simulink model "bluetooth_voice"  (Simulink 6.0)
settings: Solver=ode3  SolverMode=SingleTasking  StartTime=0.0  StopTime=2.7  RelTol=1e-3
PreLoadFcn:
  | bluetooth_init;
PostLoadFcn:
  | bluetooth_cb
values from neighbouring files (symbols this model uses):
  Access_Code = zeros(72,1); Access_Code(1:2:72)=1    [bluetooth_init.m]
  ARQ = [1]    [bluetooth_init.m]
  awgn_802_seed = randseed(3)    [bluetooth_init.m]
  awgn_channel_seed = randseed(2)    [bluetooth_init.m]
  data_seed = randseed(5)    [bluetooth_init.m]
  Flow_Control = [1]    [bluetooth_init.m]
  HV_Type = 3    [bluetooth_cb.m]
  Input_Fs = 8000    [bluetooth_init.m]
  One_Zero_Payload = zeros(240,1)    [bluetooth_init.m]
  Packet_Type = [1 0 1 0]'    [bluetooth_init.m]
  rate_802_seed = randseed(4)    [bluetooth_init.m]
  Sequence = [1]    [bluetooth_init.m]
  Slave_Address = [1 0 1]'    [bluetooth_init.m]
  Slot_Ts = (1/1600)    (= 0.000625)    [bluetooth_cb.m]
undefined symbols (not defined in the file or in its folder): figposition, Fs, jet, Num_Slots_Rate, slcm, Slot_Enable_Phase, Tx_Ts
libraries: commblkcod2 x48, dspsrcs4 x22, dspsigops x19, simulink x15, dspbuff3 x8, dspindex x7, dspsigattribs x6, dspmtrx3 x5, dsparch4 x4, commdigbbndfm2 x4, bluetooth_lib x4, dspsnks4 x4
(part 1 of 2)
CloseFcn:
  | % Clear model variables
  | clear ARQ   Access_Code   BER_Results   Flow_Control   HV_Type   Input_Fs
  | clear Num_802_packets   Num_Payload_Bits   Num_Slots_Rate   One_Zero_Payload
  | clear Packet_Type   Sequence   Slave_Address   Slot_Enable_Phase   Slot_Pair
  | clear Slot_Ts   Tx_Ts   awgn_802_seed   awgn_channel_seed   data_seed
  | clear fixed_hop_freq   hop_seed   interp_coeffs   rate_802_seed   sigin
  | clear sigout   bluetoothSigsOut   y
settings Model: Creator=Stuart McGarrity  LastModifiedBy=mmclerno  ExtModeAutoUpdateStatusClock=off  BufferReuse=off  ProdHWDeviceType=Specified
settings Model: ModifiedComment=|
  | stuartm -- Fri Jul 20 12:58:27 2001 -- Version 1.201
  | Fix for R12.1. Changed CPM modulator. Replaced enable subsystems in channel with "switch case".
settings DataIOCC: SaveOutput=off  SaveTime=off  SignalLoggingName=bluetoothSigsOut
settings OptimizationCC: BlockReduction=off  BooleanDataType=off  InlineInvariantSignals=off  OptimizeBlockIOStorage=off  BufferReuse=off  EnforceIntegerDowncast=off  ExpressionFolding=off  FoldNonRolledExpr=off  LocalBlockOutputs=off
settings DebuggingCC: SolverPrmCheckMsg=none  InheritedTsInSrcMsg=none
settings HardwareCC: ProdHWDeviceType=Specified
settings ModelReferenceCC: UpdateModelReferenceTargets=IfOutOfDate
settings CodeAppCC: MangleLength=5

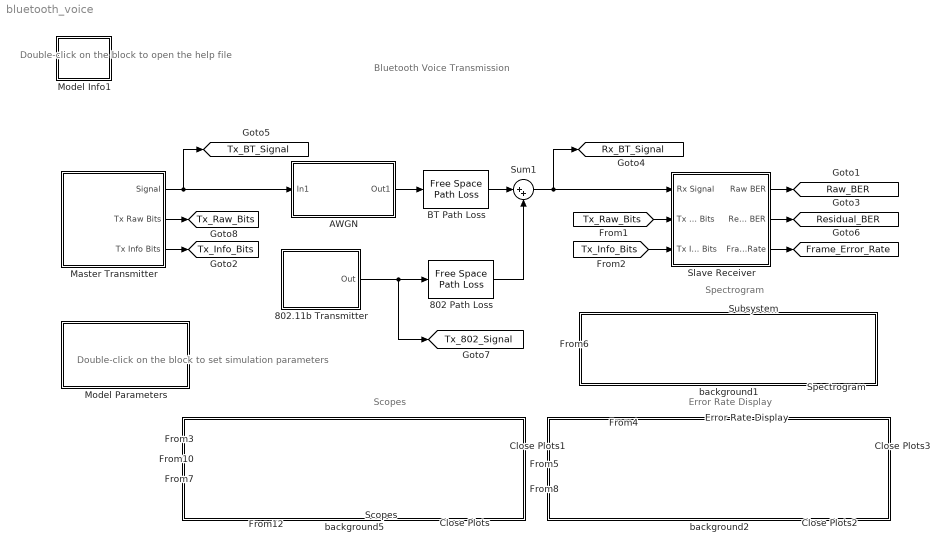
== system bluetooth_voice ==
  note: Bluetooth Voice Transmission
  note: Spectrogram
  note: Error Rate Display
  note: Scopes
  note: Double-click on the block
      | to open the help file
  note: Double-click on the block
      | to set simulation parameters
  802 Path Loss : commrflib2/Free Space Path Loss  mode=Decibels  dB=40  d=0.100  fc=1920
  802.11b Transmitter : Subsystem  AncestorBlock=bluetooth_lib/802.11b Transmitter  PropExecContextAcrossSSBoundary=on  mask{On=on, rate=200, m=1e-3, power=0.1, Freq_Number=39, rate_seed=rate_802_seed, awgn_seed=awgn_802_seed}
      mask prompts: On "Turn On 802.11"; rate "Average Rate (1/sec) (999 for constant)"; m "Length (secs)"; Freq_Number "Frequency Number (0-78)"; rate_seed "Rate Seed"; awgn_seed "Noise seed"
      mask init:
      | if On==1
      |    str='On';
      | else
      |   str='Off';
      | end;
      | 
      | adjusted_rate=rate/(1-rate*m); % account for finite packet length reducing rate
      mask Display: disp(['802.11b\nInterferer\n' str])
  AWGN : Subsystem  TreatAsAtomicUnit=on  PropExecContextAcrossSSBoundary=on  mask(Optional channel){AWGN_On=off, EsNo=15, Power=.001, Symbol_Period=1e-6, seed=awgn_channel_seed}
      mask prompts: AWGN_On "Turn on AWGN"; EsNo "Es/No"; Power "Input Power"; Symbol_Period "Symbol Period"
      mask init:
      | if AWGN_On==1
      |    Name='On';
      | else
      |   Name='Off';
      | end;
      mask Display: disp(['AWGN is ' Name])
  BT Path Loss : commrflib2/Free Space Path Loss  mode=Decibels  dB=40  d=0.100  fc=1920
  Close Plots : Subsystem  PropExecContextAcrossSSBoundary=on
      settings: OpenFcn=|
      | set_param([gcs,'/Scopes/State'],'Value','0');
      |   sdspfscope2([],[],[],'ScopeUpdate',[gcs '/Scopes/Subsystem/Timing Diagram'],'CloseFig');
      |   sdspfscope2([],[],[],'ScopeUpdate',[gcs '/Scopes/Subsystem/Spectrum Plot'],'CloseFig');
      | 
      | set_param([gcs '/Scopes/Subsystem/Timing Diagram'],'OpenScopeAtSimStart','off');
      | 
      | set_param([gcs '/Scopes/Subsystem/Spectrum Plot'],'OpenScopeAtSimStart','off');
      mask Display: disp('Close Scopes');
  Close Plots1 : Subsystem  PropExecContextAcrossSSBoundary=on
      settings: OpenFcn=|
      | set_param([gcs,'/Scopes/State'],'Value','1');
      |   sdspfscope2([],[],[],'ScopeUpdate',[gcs '/Scopes/Subsystem/Timing Diagram'],'OpenFig');
      |   sdspfscope2([],[],[],'ScopeUpdate',[gcs '/Scopes/Subsystem/Spectrum Plot'],'OpenFig');
      | 
      | set_param([gcs '/Scopes/Subsystem/Timing Diagram'],'OpenScopeAtSimStart','on');
      | 
      | set_param([gcs '/Scopes/Subsystem/Spectrum Plot'],'OpenScopeAtSimStart','on');
      mask Display: disp('Open Scopes');
  Close Plots2 : Subsystem  PropExecContextAcrossSSBoundary=on
      settings: OpenFcn=set_param([gcs '/Error Rate Display'],'Open','off');
      mask Display: disp('Close Scopes');
  Close Plots3 : Subsystem  PropExecContextAcrossSSBoundary=on
      settings: OpenFcn=set_param([gcs '/Error Rate Display'],'Open','on');
      mask Display: disp('Open Scopes');
  Error Rate Display : Subsystem  TreatAsAtomicUnit=on  PropExecContextAcrossSSBoundary=on
      mask Display: disp('Error\nRate\nDisplay')
  Master Transmitter : Subsystem  PropExecContextAcrossSSBoundary=on
      mask Type: Master Transmitter
      mask Display: plot(0,0,100,100,[30,60,60,55,55,30,30],[10,10,90,90,70,70,10],[35,35,55,55,35],[64,45,45,64,64])
  Model Info1 : Subsystem  LoadFcn=slcm LoadBlock;  InitFcn=slcm('UpdateAllCMBlocksInThisModelInit')  PropExecContextAcrossSSBoundary=on  mask(CMBlock){InitialSaveTempField=, InitialBlockCM=none, BlockCM=none, Frame=on, SaveTempField=, DisplayStringWithTags=Info, MaskDisplayString=Info, HorizontalTextAlignment=Center, LeftAlignmentValue=0.5, SourceBlockDiagram=bluetooth_voice, TagMaxNumber=20, CMTag1=, CMTag2=, CMTag3=, CMTag4=, CMTag5=, CMTag6=, CMTag7=, CMTag8=, CMTag9=, CMTag10=, CMTag11=, CMTag12=, CMTag13=, CMTag14=, CMTag15=, CMTag16=, CMTag17=, CMTag18=, CMTag19=, CMTag20=}
      mask help: This block allows revision control information to be displayed within the model.
      settings: CopyFcn=slcm CopyBlock;  DeleteFcn=slcm Cancel;  PostSaveFcn=slcm('UpdateAllCMBlocksInThisModel')  NameChangeFcn=slcm Rename;  OpenFcn=commdemohelp;
      mask Display: text(str2num(LeftAlignmentValue), 0.5, MaskDisplayString, 'HorizontalAlignment', HorizontalTextAlignment)
  Model Parameters : Subsystem  TreatAsAtomicUnit=on  PropExecContextAcrossSSBoundary=on  mask(Bluetooth Initial Settings ){HV_Type=HV3, Slot_Pair1=1&2, Slot_Pair2=5&6}
      mask prompts: HV_Type "HV Packet Type"; Slot_Pair1 "Initial Slot Pair for HV2"; Slot_Pair2 "Initial Slot Pair for HV3"
      mask help: Use the following mask to select different parameters for simulation.
      mask StyleString: popup(HV1|HV2|HV3),popup(1&2|3&4),popup(1&2|3&4|5&6)
      mask CallbackString: bluetooth_cb;||
      mask Display: disp('Double-click\n to select\n Model Parameters')
  Scopes : Subsystem  TreatAsAtomicUnit=on  PropExecContextAcrossSSBoundary=on
      mask Display: disp('Scopes')
  Slave Receiver : Subsystem  PropExecContextAcrossSSBoundary=on
      mask Type: Slave Receiver
      mask Display: plot(15,5,95,80,[26, 28,35,44,58,85,87,92,86,59,46,46,38, 31, 27,26],[55,49,45,45,34,15,10,16,17,37,50,58,66,67,62,55],[32,34,37,42,46,46],[67,69,71,70,66,58],[27,25,24,21,23,26],[52,49,45,47,52,58],[35,38,40,42,44],[66,67,66,64,61],[34,32,38,40,34],[60,56,51,55,60])
  Spectrogram : dspsnks4/Matrix Viewer  ImageParams=on  CMapStr=jet(256)  AxisColorbar=off  AxisParams=on  AxisOrigin=Lower left corner  XLabel=Time Index  YLabel=Frequency Index  ZLabel=dB Magnitude  FigPos=figposition([2.5 8.5 70 25]);  AxisZoom=on
      settings: YMin=-60  YMax=-30
  Subsystem : Subsystem  PropExecContextAcrossSSBoundary=on
      mask Display: disp('Rx_BT_Signal\nProcessing')
  Sum1 : Sum  Inputs=|++  SaturateOnIntegerOverflow=on  InputSameDT=on
  background1 : Subsystem  PropExecContextAcrossSSBoundary=on
      mask Display: disp('')
  background2 : Subsystem  PropExecContextAcrossSSBoundary=on
      mask Display: disp('')
  background5 : Subsystem  PropExecContextAcrossSSBoundary=on
      mask Display: disp('')
  tag scope: Frame_Error_Rate=global, Raw_BER=global, Residual_BER=global, Rx_BT_Signal=global, Tx_802_Signal=global, Tx_BT_Signal=global, Tx_Info_Bits=global, Tx_Raw_Bits=global
  wires:
  Sum1/1 -> [Rx_BT_Signal], Slave Receiver/1(Rx Signal)
  Master Transmitter/2(Tx Raw Bits) -> [Tx_Raw_Bits]
  [Tx_Raw_Bits] -> Slave Receiver/2(Tx Raw Bits)
  Master Transmitter/3(Tx Info Bits) -> [Tx_Info_Bits]
  [Tx_Info_Bits] -> Slave Receiver/3(Tx Info Bits)
  802.11b Transmitter/1(Out) -> [Tx_802_Signal], 802 Path Loss/1
  802 Path Loss/1 -> Sum1/2
  AWGN/1(Out1) -> BT Path Loss/1
  BT Path Loss/1 -> Sum1/1
  [Tx_BT_Signal] -> Scopes/1(Tx)
  [Rx_BT_Signal] -> Scopes/3(Rx)
  [Tx_802_Signal] -> Scopes/2(Tx_802)
  [Packet_Envelope_802] -> Scopes/4(Tx_802 Envelope)
  Master Transmitter/1(Signal) -> AWGN/1(In1), [Tx_BT_Signal]
  Slave Receiver/1(Raw BER) -> [Raw_BER]
  Slave Receiver/2(Residual BER) -> [Residual_BER]
  Slave Receiver/3(Frame Error Rate) -> [Frame_Error_Rate]
  [Raw_BER] -> Error Rate Display/1(Tx)
  [Residual_BER] -> Error Rate Display/2(Tx_802)
  [Frame_Error_Rate] -> Error Rate Display/3(Rx)
  Subsystem/1(Out1) -> Spectrogram/1
  [Rx_BT_Signal] -> Subsystem/1(In1)

== system bluetooth_voice/802.11b Transmitter ==
  1/100packet resolution : ZeroOrderHold  SampleTime=(1/1600)/100
  22MHz noise in 100MHz signal : Subsystem  TreatAsAtomicUnit=on  PropExecContextAcrossSSBoundary=on
  Buffer to same frame-size as channel : dspbuff3/Buffer  N=62500  V=0  ic=0
  Enable control : Subsystem  PropExecContextAcrossSSBoundary=on
      mask Display:
      | disp('Enable\n
      | Logic')
  Square pulse with Poisson process : Subsystem  PropExecContextAcrossSSBoundary=on  mask(Poisson process){rate=adjusted_rate, m=m, seed=rate_seed}
      mask prompts: rate "Average Rate (1/sec)"; m "Mean Length"
      mask Display: plot(exp(-(0:.4:3)))
  Out : Outport
  tag scope: Packet_Envelope_802=global
  wires:
  22MHz noise in 100MHz signal/1(Out) -> Buffer to same frame-size as channel/1
  Buffer to same frame-size as channel/1 -> Out/1
  1/100packet resolution/1 -> Enable control/1(In)
  Square pulse with Poisson process/1(hit) -> 1/100packet resolution/1, [Packet_Envelope_802]
  Enable control/1(Out) -> 22MHz noise in 100MHz signal/Enable

== system bluetooth_voice/AWGN ==
  In1 : Inport  LatchInput=off
  Generate noise only for slot 1 : simulink/Signal Routing/Manual Switch  sw=0  action=0
  Mode : Constant  Value=AWGN_On  SampleTime=Inf
  Slot 1 enable2 : dspsrcs4/Signal From Workspace  X=[1 0 0 0 0 0]  Ts=625e-6  nsamps=1  OutputAfterFinalValue=Cyclic repetition
  Slot 1 enable3 : dspsrcs4/Signal From Workspace  X=[1 1 1 1 1 1 ]  Ts=625e-6  nsamps=1  OutputAfterFinalValue=Cyclic repetition
  Subsystem : Subsystem  TreatAsAtomicUnit=on  PropExecContextAcrossSSBoundary=on
  Out1 : Outport  InitialOutput=0
  wires:
  Mode/1 -> Subsystem/1(In1)
  Subsystem/1(Out1) -> Out1/1
  Slot 1 enable3/1 -> Generate noise only for slot 1/2
  Generate noise only for slot 1/1 -> Subsystem/Enable
  Slot 1 enable2/1 -> Generate noise only for slot 1/1
  In1/1 -> Subsystem/2(In2)

== system bluetooth_voice/Close Plots ==

== system bluetooth_voice/Close Plots1 ==

== system bluetooth_voice/Close Plots2 ==

== system bluetooth_voice/Close Plots3 ==

== system bluetooth_voice/Error Rate Display ==
  note: Total number of bits
  note: Raw Bit Errors
  note: Raw BER
  note: Residual BER
  note: Residual Bit Error
  note: Total number of bits
  note: FER
  note: Frame Errors
  note: Total number of Frames
  Tx : Inport  LatchInput=off
  Tx_802 : Inport  Port=2  LatchInput=off
  Rx : Inport  Port=3  LatchInput=off
  FER Display : Display
  Raw BER Display : Display
  Residual BER Display : Display
  wires:
  Rx/1 -> FER Display/1
  Tx/1 -> Raw BER Display/1
  Tx_802/1 -> Residual BER Display/1

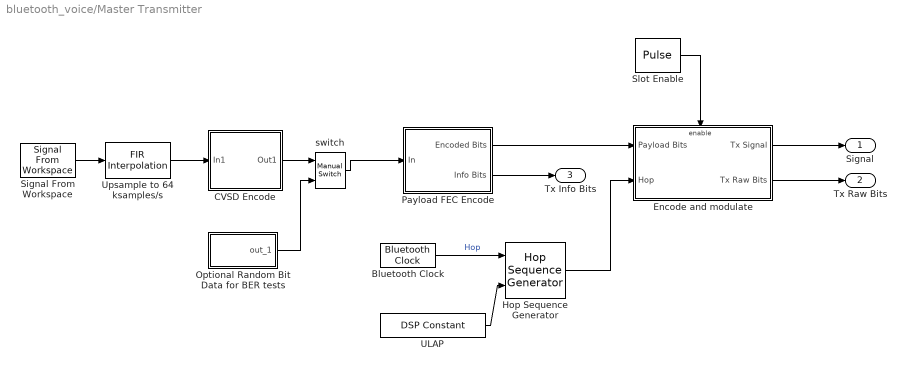
== system bluetooth_voice/Master Transmitter ==
  Bluetooth Clock : bluetooth_lib/Bluetooth Clock  Ts=(1/1600)/2
  CVSD Encode : Subsystem  PropExecContextAcrossSSBoundary=on  mask(CVSD Encoder){min_step=10, max_step=1280, accum_decay=1-1/32, step_decay=1-1/1024}
      mask prompts: min_step "Minimum Step Size"; max_step "Maximum Step Size"; accum_decay "Accumulator Decay"; step_decay "Step Decay"
      mask help: Encode a 64 K samples per sec speech signal into a 64Kbps bit stream.
      mask init:
      | pos_accum_max = 2^15 - 1;
      | neg_accum_max = -2^15 + 1;
      mask Display: disp('CVSD\nEncode')
  Encode and modulate : Subsystem  TreatAsAtomicUnit=on  PropExecContextAcrossSSBoundary=on
  Hop Sequence Generator : bluetooth_lib/Hop Sequence Generator  Hop_Mode=Connection State Hop Sequence  hop_seed=hop_seed  fixed_hop_freq=fixed_hop_freq
  Optional Random Bit Data for BER tests : Subsystem  PropExecContextAcrossSSBoundary=on  mask(Random-Integer Generator){mul=2, seed=data_seed, Ts=1/64000, frameBased=off, sampPerFrame=1, orient=off}
      mask prompts: mul "M-ary number:"; seed "Initial seed:"; Ts "Sample time:"; frameBased "Frame-based outputs"; sampPerFrame "Samples per frame:"; orient "Interpret vector parameters as 1-D"
      mask help: Generate integers randomly distributed in range [0, M-1], where M is the M-ary number.
      mask init:
      | if (frameBased & sampPerFrame > 1), dsp_sampFrame = sampPerFrame;
      | else dsp_sampFrame = 1; end
      | eStr=commblkrandintsrc2(gcb,'init');
      | if(eStr.ecode==1)
      |     error(eStr.emsg);
      | end
      mask Help: helpview(commbhelp)
      mask CallbackString: |||commblkrandintsrc2(gcb,'cbFrameBased');||commblkrandintsrc2(gcb,'cbOrient');
      mask Display: disp('Random bits')
  Payload FEC Encode : Subsystem  PropExecContextAcrossSSBoundary=on
  Signal From Workspace : dspsrcs4/Signal From Workspace  X=sigin  Ts=1/8000  nsamps=1  OutputAfterFinalValue=Setting to zero
  Slot Enable : DiscretePulseGenerator  Period=Num_Slots_Rate  PhaseDelay=Slot_Enable_Phase  SampleTime=Slot_Ts
  ULAP : dspsrcs4/DSP Constant  Value=hex2dec('2a96ef25')  SampleMode=Discrete  discreteOutput=Sample-based  continuousOutput=Sample-based  sampTime=(1/1600)/2  framePeriod=(1/1600)/2  dataType=Inherit from 'Constant value'  isSigned=on  wordLen=16  udDataType=sfix(16)  fracBitsMode=Best precision  numFracBits=15  InterpretAs1D=off  Ts=(1/1600)/2  FramebasedOutput=off
  Upsample to 64 ksamples/s : dspmlti3/FIR Interpolation  DialogController=dspDDGCreate  DialogControllerArgs=DataTag4  h=interp_coeffs  L=8  framing=Maintain input frame size  outputBufInitCond=0  roundingMode=Floor  overflowMode=off
  switch : simulink/Signal Routing/Manual Switch  sw=1  action=0
  Signal : Outport
  Tx Raw Bits : Outport  Port=2
  Tx Info Bits : Outport  Port=3
  wires:
  Slot Enable/1 -> Encode and modulate/Enable
  Encode and modulate/1(Tx Signal) -> Signal/1
  Payload FEC Encode/1(Encoded Bits) -> Encode and modulate/1(Payload Bits)
  Signal From Workspace/1 -> Upsample to 64 ksamples/s/1
  Payload FEC Encode/2(Info Bits) -> Tx Info Bits/1
  Encode and modulate/2(Tx Raw Bits) -> Tx Raw Bits/1
  Hop Sequence Generator/1 -> Encode and modulate/2(Hop)
  ULAP/1 -> Hop Sequence Generator/2
  Bluetooth Clock/1 -> Hop Sequence Generator/1  "Hop"
  Optional Random Bit Data for BER tests/1(out_1) -> switch/2
  CVSD Encode/1(Out1) -> switch/1
  switch/1 -> Payload FEC Encode/1(In)
  Upsample to 64 ksamples/s/1 -> CVSD Encode/1(In1)

== system bluetooth_voice/Model Info1 ==
  EmptySubsystem : Subsystem  PropExecContextAcrossSSBoundary=on

== system bluetooth_voice/Model Parameters ==

== system bluetooth_voice/Scopes ==
  Tx : Inport  LatchInput=off
  Tx_802 : Inport  Port=2  LatchInput=off
  Rx : Inport  Port=3  LatchInput=off
  Tx_802 Envelope : Inport  Port=4  LatchInput=off
  802.11 Packets  Transmitted : Display
  Counter : dspswit3/Counter  Direction=Up  CountEvent=Rising edge  CounterSize=User defined  MaxCount=1000  InitialCount=0  Output=Count  HitValue=32  ResetInput=off  SamplesPerFrame=1  Ts=1  CntDtype=double  HitDtype=Logical
  State : Constant
  Subsystem : Subsystem  TreatAsAtomicUnit=on  PropExecContextAcrossSSBoundary=on
  To Workspace : ToWorkspace  VariableName=Num_802_packets  SampleTime=-1  SaveFormat=Array
      settings: MaxDataPoints=1
  wires:
  Counter/1 -> To Workspace/1, 802.11 Packets  Transmitted/1
  State/1 -> Subsystem/Enable
  Tx_802 Envelope/1 -> Counter/1
  Tx_802/1 -> Subsystem/2(In2)
  Tx/1 -> Subsystem/1(In1)
  Rx/1 -> Subsystem/3(In3)

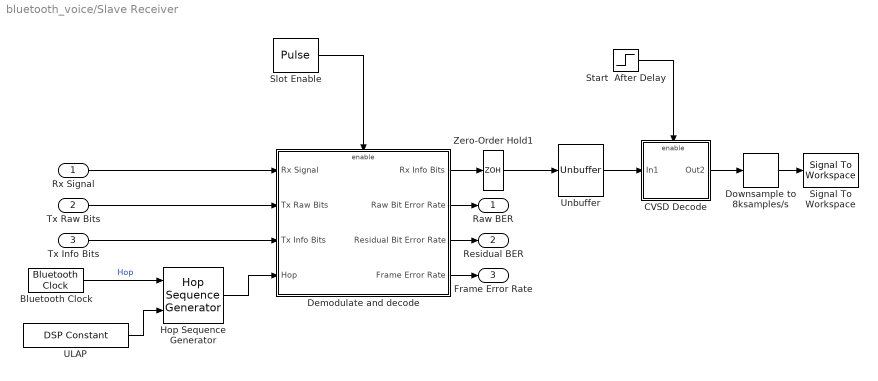
== system bluetooth_voice/Slave Receiver ==
  Rx Signal : Inport  LatchInput=off
  Tx Raw Bits : Inport  Port=2  LatchInput=off
  Tx Info Bits : Inport  Port=3  LatchInput=off
  Bluetooth Clock : bluetooth_lib/Bluetooth Clock  Ts=(1/1600)/2
  CVSD Decode : Subsystem  TreatAsAtomicUnit=on  PropExecContextAcrossSSBoundary=on  mask(CVSD Decoder){min_step=10, max_step=1280, accum_decay=1-1/32, step_decay=1-1/1024}
      mask prompts: min_step "Minimum Step Size"; max_step "Maximum Step Size"; accum_decay "Accumulator Decay"; step_decay "Step Decay"
      mask init:
      | pos_accum_max = 2^15 - 1;
      | neg_accum_max = -2^15 + 1;
      mask Display: disp('CVSD\nDecoder')
  Demodulate and decode : Subsystem  TreatAsAtomicUnit=on  PropExecContextAcrossSSBoundary=on
  Downsample to 8ksamples/s : dspsigops/Downsample  N=8  phase=0  ic=0  smode=Allow multirate  fmode=Maintain input frame size
  Hop Sequence Generator : bluetooth_lib/Hop Sequence Generator  Hop_Mode=Connection State Hop Sequence  hop_seed=hop_seed  fixed_hop_freq=fixed_hop_freq
  Signal To Workspace : dspsnks4/Signal To Workspace  VariableName=sigout  FrameMode=Concatenate frames (2-D array)
      settings: FixptAsFi=off
  Slot Enable : DiscretePulseGenerator  Period=Num_Slots_Rate  PhaseDelay=Slot_Enable_Phase  SampleTime=Slot_Ts
  Start  After Delay : Step  Time=0.01  SampleTime=1/64000
  ULAP : dspsrcs4/DSP Constant  Value=hex2dec('2a96ef25')  SampleMode=Discrete  discreteOutput=Sample-based  continuousOutput=Sample-based  sampTime=(1/1600)/2  framePeriod=(1/1600)/2  dataType=Inherit from 'Constant value'  isSigned=on  wordLen=16  udDataType=sfix(16)  fracBitsMode=Best precision  numFracBits=15  InterpretAs1D=off  Ts=(1/1600)/2  FramebasedOutput=off
  Unbuffer : dspbuff3/Unbuffer  ic=0
  Zero-Order Hold1 : ZeroOrderHold  SampleTime=Tx_Ts
  Raw BER : Outport  InitialOutput=0
  Residual BER : Outport  Port=2  InitialOutput=0
  Frame Error Rate : Outport  Port=3  InitialOutput=0
  wires:
  Slot Enable/1 -> Demodulate and decode/Enable
  Rx Signal/1 -> Demodulate and decode/1(Rx Signal)
  Tx Raw Bits/1 -> Demodulate and decode/2(Tx Raw Bits)
  CVSD Decode/1(Out2) -> Downsample to 8ksamples/s/1
  Demodulate and decode/1(Rx Info Bits) -> Zero-Order Hold1/1
  ULAP/1 -> Hop Sequence Generator/2
  Bluetooth Clock/1 -> Hop Sequence Generator/1  "Hop"
  Hop Sequence Generator/1 -> Demodulate and decode/4(Hop)
  Zero-Order Hold1/1 -> Unbuffer/1
  Start  After Delay/1 -> CVSD Decode/Enable
  Unbuffer/1 -> CVSD Decode/1(In1)
  Tx Info Bits/1 -> Demodulate and decode/3(Tx Info Bits)
  Demodulate and decode/3(Residual Bit Error Rate) -> Residual BER/1
  Demodulate and decode/2(Raw Bit Error Rate) -> Raw BER/1
  Demodulate and decode/4(Frame Error Rate) -> Frame Error Rate/1
  Downsample to 8ksamples/s/1 -> Signal To Workspace/1

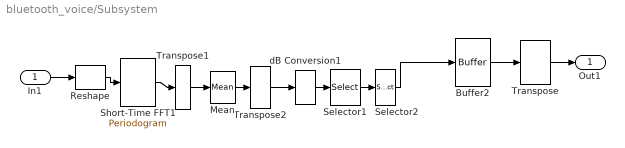
== system bluetooth_voice/Subsystem ==
  In1 : Inport  LatchInput=off
  Buffer2 : dspbuff3/Buffer  N=60  V=59  ic=-70
  Mean : dspstat3/Mean  DialogController=dspDDGCreate  DialogControllerArgs=DataTag8  run=off  reset_popup=None  roundingMode=Floor  overflowMode=off
  Reshape : simulink/Math Operations/Reshape  OutputDimensionality=Customize  OutputDimensions=[500,125]
  Selector1 : Selector  Elements=[257:512 1:256]  InputPortWidth=512
  Selector2 : Selector  Elements=7:506  InputPortWidth=512
  Short-Time FFT1 : dspspect3/Periodogram  wintype=Hanning  Rs=50  beta=5  winsamp=Periodic  inheritFFT=off  fftsize=512  navg=1
  Transpose : dspmtrx3/Transpose  Hermitian=off  overflowFlag=on
  Transpose1 : dspmtrx3/Transpose  Hermitian=off  overflowFlag=on
  Transpose2 : dspmtrx3/Transpose  Hermitian=off  overflowFlag=on
  dB Conversion1 : dspmathops/dB Conversion  dBtype=dB  intype=Power  R=1  fuzz=on
  Out1 : Outport
  wires:
  Selector2/1 -> Buffer2/1
  Selector1/1 -> Selector2/1
  Buffer2/1 -> Transpose/1
  Transpose2/1 -> dB Conversion1/1
  Transpose1/1 -> Mean/1
  Mean/1 -> Transpose2/1
  Reshape/1 -> Short-Time FFT1/1
  Short-Time FFT1/1 -> Transpose1/1
  dB Conversion1/1 -> Selector1/1
  Transpose/1 -> Out1/1
  In1/1 -> Reshape/1

== system bluetooth_voice/background1 ==

== system bluetooth_voice/background2 ==

== system bluetooth_voice/background5 ==

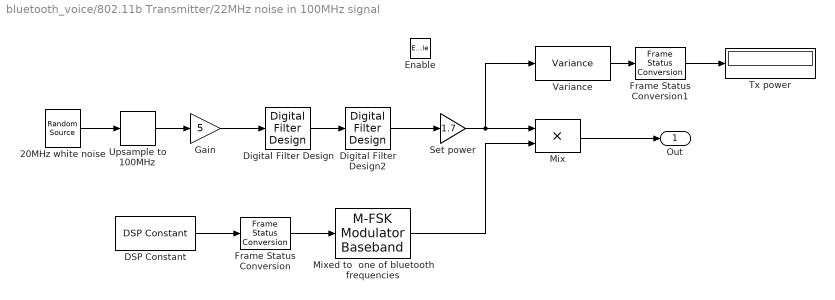
== system bluetooth_voice/802.11b Transmitter/22MHz noise in 100MHz signal ==
  Enable : EnablePort
  20MHz white noise : dspsrcs4/Random Source  SrcType=Gaussian  NormMethod=Ziggurat  CltLength=12  Min=0  Max=1  Mean=0  Var=power  RepMode=Specify seed  rawSeed=awgn_seed  Inherit=off  SampMode=Discrete  SampTime=1/20e6  SampFrame=62500/500  DataType=Double  OutComplex=Complex
  DSP Constant : dspsrcs4/DSP Constant  Value=Freq_Number  SampleMode=Discrete  discreteOutput=Sample-based  continuousOutput=Sample-based  sampTime=.01/1600  framePeriod=.01/1600  dataType=Inherit from 'Constant value'  isSigned=on  wordLen=16  udDataType=sfix(16)  fracBitsMode=Best precision  numFracBits=15  InterpretAs1D=off  Ts=.01/1600  FramebasedOutput=off
  Digital Filter Design : dsparch4/Digital Filter Design
  Digital Filter Design2 : dsparch4/Digital Filter Design
  Frame Status Conversion : dspsigattribs/Frame Status Conversion  growRefPort=off  outframe=Frame-based
  Frame Status Conversion1 : dspsigattribs/Frame Status Conversion  growRefPort=off  outframe=Sample-based
  Gain : Gain  Gain=5  SaturateOnIntegerOverflow=on
  Mix : Product  SaturateOnIntegerOverflow=on  InputSameDT=on
  "Mixed to  one of bluetooth frequencies " : commdigbbndfm2/M-FSK Modulator Baseband  M=79  InType=Integer  Enc=Binary  freqSep=1e6  phaseType=Continuous  numSamp=6.25e4/100
  Set power : Gain  Gain=1.7  SaturateOnIntegerOverflow=on
  Tx power : Display
  Upsample to 100MHz : dspsigops/Upsample  N=5  phase=0  ic=0  mode=Maintain input frame rate
  Variance : dspstat3/Variance  DialogController=dspDDGCreate  DialogControllerArgs=DataTag3  run=off  reset_popup=None  roundingMode=Floor  overflowMode=off
  Out : Outport  OutputWhenDisabled=reset  InitialOutput=0
  wires:
  Upsample to 100MHz/1 -> Gain/1
  Mix/1 -> Out/1
  20MHz white noise/1 -> Upsample to 100MHz/1
  Frame Status Conversion/1 -> "Mixed to  one of bluetooth frequencies "/1
  "Mixed to  one of bluetooth frequencies "/1 -> Mix/2
  DSP Constant/1 -> Frame Status Conversion/1
  Gain/1 -> Digital Filter Design/1
  Variance/1 -> Frame Status Conversion1/1
  Frame Status Conversion1/1 -> Tx power/1
  Set power/1 -> Mix/1, Variance/1
  Digital Filter Design2/1 -> Set power/1
  Digital Filter Design/1 -> Digital Filter Design2/1

== system bluetooth_voice/802.11b Transmitter/Enable control ==
  In : Inport  LatchInput=off
  If rate set to 999 turn-on always : RelationalOperator  Operator===  InputSameDT=on
  Logical Operator : Logic
  Logical Operator1 : Logic
  Logical Operator2 : Logic  Operator=OR
  Mode : Constant  Value=On
  Mode1 : Constant  Value=rate
  Mode2 : Constant  Value=999
  Out : Outport
  wires:
  Mode2/1 -> If rate set to 999 turn-on always/2
  Mode1/1 -> If rate set to 999 turn-on always/1
  If rate set to 999 turn-on always/1 -> Logical Operator1/2
  Logical Operator/1 -> Logical Operator2/1
  Mode/1 -> Logical Operator/2, Logical Operator1/1
  Logical Operator1/1 -> Logical Operator2/2
  In/1 -> Logical Operator/1
  Logical Operator2/1 -> Out/1

== system bluetooth_voice/802.11b Transmitter/Square pulse with Poisson process ==
  Abs : Abs  SaturateOnIntegerOverflow=on
  Derivative : Derivative
  Poisson Integer Generator : commrandsrc2/Poisson Integer Generator  lambda=adjusted_rate*m  seed=rate_seed  Ts=m  frameBased=off  sampPerFrame=1  orient=off
  Saturation : Saturate  UpperLimit=1  LowerLimit=0
  Zero-Order Hold : ZeroOrderHold  SampleTime=1e-3
  hit : Outport  InitialOutput=0
  wires:
  Poisson Integer Generator/1 -> Derivative/1
  Derivative/1 -> Saturation/1
  Abs/1 -> Zero-Order Hold/1
  Saturation/1 -> Abs/1
  Zero-Order Hold/1 -> hit/1

== system bluetooth_voice/AWGN/Subsystem ==
  In1 : Inport  LatchInput=off
  In2 : Inport  Port=2  LatchInput=off
  Enable : EnablePort
  Add noise : Subsystem  TreatAsAtomicUnit=on  PropExecContextAcrossSSBoundary=on
  If : If  IfExpression=u1 == 0
  Merge : Merge
  Pass Through : Subsystem  TreatAsAtomicUnit=on  PropExecContextAcrossSSBoundary=on
  Out1 : Outport
  wires:
  Add noise/1(Out1) -> Merge/2
  Pass Through/1(Out1) -> Merge/1
  If/1 -> Pass Through/Action
  In2/1 -> Pass Through/1(In1), Add noise/1(In1)
  If/2 -> Add noise/Action
  In1/1 -> If/1
  Merge/1 -> Out1/1

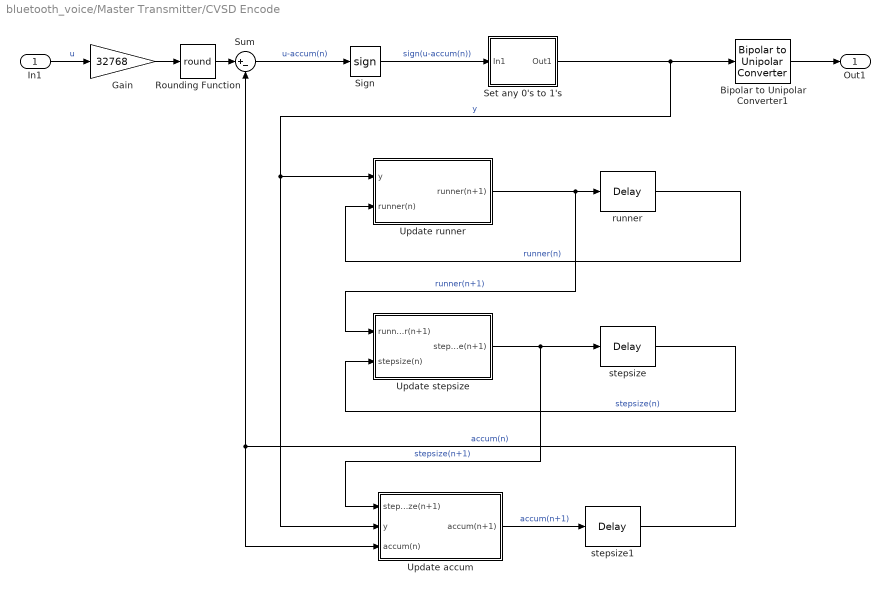
== system bluetooth_voice/Master Transmitter/CVSD Encode ==
  In1 : Inport  LatchInput=off
  Bipolar to Unipolar Converter1 : commutil2/Bipolar to Unipolar Converter  M=2  polarity=Negative
  Gain : Gain  Gain=32768  SaturateOnIntegerOverflow=on
  Rounding Function : Rounding  Operator=round
  Set any 0's to 1's : Subsystem  PropExecContextAcrossSSBoundary=on
  Sign : Signum
  Sum : Sum  Inputs=|+-  SaturateOnIntegerOverflow=on  InputSameDT=on
  Update accum : Subsystem  PropExecContextAcrossSSBoundary=on
  Update runner : Subsystem  PropExecContextAcrossSSBoundary=on
  Update stepsize : Subsystem  PropExecContextAcrossSSBoundary=on
  runner : dspsigops/Delay  dly_unit=Samples  delay=1  ic_detail=on  dif_ic_for_ch=off  dif_ic_for_dly=off  ic=10  reset_popup=None
  stepsize : dspsigops/Delay  dly_unit=Samples  delay=1  ic_detail=on  dif_ic_for_ch=off  dif_ic_for_dly=off  ic=min_step  reset_popup=None
  stepsize1 : dspsigops/Delay  dly_unit=Samples  delay=1  ic_detail=on  dif_ic_for_ch=off  dif_ic_for_dly=off  ic=min_step  reset_popup=None
  Out1 : Outport
  wires:
  Gain/1 -> Rounding Function/1
  Rounding Function/1 -> Sum/1
  Bipolar to Unipolar Converter1/1 -> Out1/1
  In1/1 -> Gain/1  "u"
  Sum/1 -> Sign/1  "u-accum(n)"
  stepsize1/1 -> Sum/2, Update accum/3(accum(n))  "accum(n)"
  Set any 0's to 1's/1(Out1) -> Bipolar to Unipolar Converter1/1, Update runner/1(y), Update accum/2(y)  "y"
  runner/1 -> Update runner/2(runner(n))  "runner(n)"
  Update runner/1(runner(n+1)) -> Update stepsize/1(runner(n+1)), runner/1  "runner(n+1)"
  Sign/1 -> Set any 0's to 1's/1(In1)  "sign(u-accum(n))"
  stepsize/1 -> Update stepsize/2(stepsize(n))  "stepsize(n)"
  Update stepsize/1(stepsize(n+1)) -> Update accum/1(stepsize(n+1)), stepsize/1  "stepsize(n+1)"
  Update accum/1(accum(n+1)) -> stepsize1/1  "accum(n+1)"

== system bluetooth_voice/Master Transmitter/Encode and modulate ==
  note: Framing: Bluetooth spec page 47
      | HEC: Bluetooth spec page 72
  Payload Bits : Inport  SampleTime=625e-6  LatchInput=off
  Hop : Inport  Port=2  SampleTime=625e-6  LatchInput=off
  Enable : EnablePort
  Access Code : dspsrcs4/DSP Constant  Value=Access_Code  SampleMode=Discrete  discreteOutput=Frame-based  continuousOutput=Sample-based  sampTime=Slot_Ts  framePeriod=Slot_Ts  dataType=Inherit from 'Constant value'  isSigned=on  wordLen=16  udDataType=sfix(16)  fracBitsMode=Best precision  numFracBits=15  InterpretAs1D=off  Ts=Slot_Ts  FramebasedOutput=on
  "Concatenate Access, Header and Payload" : simulink/Math Operations/Matrix Concatenation  numInports=3  catMethod=Vertical
  GFSK Modulate and frequency hop : Subsystem  PropExecContextAcrossSSBoundary=on
  General CRC Generator : commcrc2/General CRC Generator  genPoly=[1 1 0 1 0 0 1 1 1]  iniStates=[1 0 0 1 0 1 1 0]  numChecksums=1
  Header Info : Subsystem  PropExecContextAcrossSSBoundary=on
      mask Display: disp('Header Info')
  Header Info FEC Encode : dspsigops/Repeat  N=3  ic=0  mode=Maintain input frame rate
  Tx Signal : Outport  OutputWhenDisabled=reset  InitialOutput=0
  Tx Raw Bits : Outport  Port=2  OutputWhenDisabled=reset  InitialOutput=0
  wires:
  GFSK Modulate and frequency hop/1(Tx SIgnal) -> Tx Signal/1
  "Concatenate Access, Header and Payload"/1 -> GFSK Modulate and frequency hop/1(Tx Raw Bits), Tx Raw Bits/1
  General CRC Generator/1 -> Header Info FEC Encode/1  "HEC"
  Header Info/1(Out) -> General CRC Generator/1  "Header Info"
  Header Info FEC Encode/1 -> "Concatenate Access, Header and Payload"/2  "Header"
  Access Code/1 -> "Concatenate Access, Header and Payload"/1  "Access Code"
  Payload Bits/1 -> "Concatenate Access, Header and Payload"/3
  Hop/1 -> GFSK Modulate and frequency hop/2(Hop)

== system bluetooth_voice/Master Transmitter/Optional Random Bit Data for BER tests ==
  Frame Status Conversion : dspsigattribs/Frame Status Conversion  growRefPort=off  outframe=Sample-based
  Random Source : dspsrcs4/Random Source  SrcType=Uniform  NormMethod=Ziggurat  CltLength=12  Min=-1+eps  Max=mul-1  Mean=0  Var=1  RepMode=Specify seed  rawSeed=seed  Inherit=off  SampMode=Discrete  SampTime=Ts  SampFrame=dsp_sampFrame  DataType=Double  OutComplex=Real
  Reshape : simulink/Math Operations/Reshape  OutputDimensionality=1-D array  OutputDimensions=[sampPerFrame,max([length(mul), length(seed)])]
  Rounding Function : Rounding  Operator=ceil
  out_1 : Outport  InitialOutput=0
  wires:
  Frame Status Conversion/1 -> Reshape/1
  Random Source/1 -> Rounding Function/1
  Reshape/1 -> out_1/1
  Rounding Function/1 -> Frame Status Conversion/1

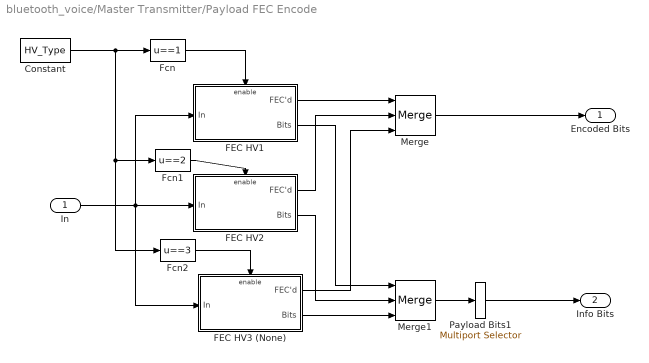
== system bluetooth_voice/Master Transmitter/Payload FEC Encode ==
  In : Inport  LatchInput=off
  Constant : Constant  Value=HV_Type
  FEC HV1 : Subsystem  TreatAsAtomicUnit=on  PropExecContextAcrossSSBoundary=on
  FEC HV2 : Subsystem  TreatAsAtomicUnit=on  PropExecContextAcrossSSBoundary=on
  FEC HV3 (None) : Subsystem  TreatAsAtomicUnit=on  PropExecContextAcrossSSBoundary=on
  Fcn : Fcn  Expr=u==1
  Fcn1 : Fcn  Expr=u==2
  Fcn2 : Fcn  Expr=u==3
  Merge : Merge  Inputs=3
  Merge1 : Merge  Inputs=3
  Payload Bits1 : dspindex/Multiport Selector  rowsOrCols=Rows  idxCellArray={1:Num_Payload_Bits}  idxErrMode=Clip Index
  Encoded Bits : Outport
  Info Bits : Outport  Port=2
  wires:
  In/1 -> FEC HV2/1(In), FEC HV1/1(In), FEC HV3 (None)/1(In)
  Constant/1 -> Fcn/1, Fcn1/1, Fcn2/1
  Fcn/1 -> FEC HV1/Enable
  Fcn1/1 -> FEC HV2/Enable
  Fcn2/1 -> FEC HV3 (None)/Enable
  FEC HV2/1(FEC'd) -> Merge/2
  FEC HV1/2(Bits) -> Merge1/1
  FEC HV2/2(Bits) -> Merge1/2
  FEC HV1/1(FEC'd) -> Merge/1
  Merge/1 -> Encoded Bits/1
  Merge1/1 -> Payload Bits1/1
  FEC HV3 (None)/1(FEC'd) -> Merge/3
  FEC HV3 (None)/2(Bits) -> Merge1/3
  Payload Bits1/1 -> Info Bits/1

== system bluetooth_voice/Model Info1/EmptySubsystem ==

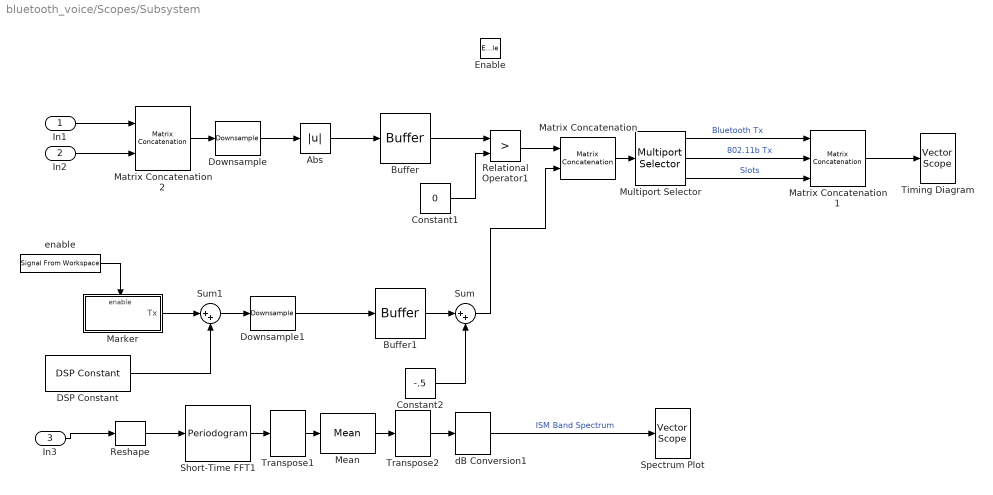
== system bluetooth_voice/Scopes/Subsystem ==
  In1 : Inport  LatchInput=off
  In2 : Inport  Port=2  LatchInput=off
  In3 : Inport  Port=3  LatchInput=off
  Enable : EnablePort
  Abs : Abs  SaturateOnIntegerOverflow=on
  Buffer : dspbuff3/Buffer  N=60*500  V=59*500  ic=0
  Buffer1 : dspbuff3/Buffer  N=60*500  V=59*500  ic=0
  Constant1 : Constant  Value=0
  Constant2 : Constant  Value=-.5
  DSP Constant : dspsrcs4/DSP Constant  Value=.2*[ones(1,36600) zeros(1,62500-36600)]'  SampleMode=Discrete  discreteOutput=Frame-based  continuousOutput=Sample-based  sampTime=625e-6  framePeriod=625e-6  dataType=Inherit from 'Constant value'  isSigned=on  wordLen=16  udDataType=sfix(16)  fracBitsMode=Best precision  numFracBits=15  InterpretAs1D=off  Ts=625e-6  FramebasedOutput=on
  Downsample : dspsigops/Downsample  N=125  phase=0  ic=0  smode=Allow multirate  fmode=Maintain input frame rate
  Downsample1 : dspsigops/Downsample  N=125  phase=0  ic=0  smode=Allow multirate  fmode=Maintain input frame rate
  Marker : Subsystem  TreatAsAtomicUnit=on  PropExecContextAcrossSSBoundary=on
  Matrix Concatenation : simulink/Math Operations/Matrix Concatenation  numInports=2  catMethod=Horizontal
  Matrix Concatenation1 : simulink/Math Operations/Matrix Concatenation  numInports=3  catMethod=Horizontal
  Matrix Concatenation2 : simulink/Math Operations/Matrix Concatenation  numInports=2  catMethod=Horizontal
  Mean : dspstat3/Mean  DialogController=dspDDGCreate  DialogControllerArgs=DataTag5  run=off  reset_popup=None  roundingMode=Floor  overflowMode=off
  Multiport Selector : dspindex/Multiport Selector  rowsOrCols=Columns  idxCellArray={ 1,2,3}  idxErrMode=Clip Index
  Relational Operator1 : RelationalOperator  Operator=>  InputSameDT=on
  Reshape : simulink/Math Operations/Reshape  OutputDimensionality=Customize  OutputDimensions=[500,125]
  Short-Time FFT1 : dspspect3/Periodogram  wintype=Hanning  Rs=50  beta=5  winsamp=Periodic  inheritFFT=off  fftsize=512  navg=1
  Spectrum Plot : dspsnks4/Vector Scope  ScopeProperties=off  Domain=Frequency  HorizSpan=1  DisplayProperties=off  AxisGrid=on  Memory=off  FrameNumber=on  AxisLegend=on  AxisZoom=off  OpenScopeAtSimStart=on  OpenScopeImmediately=off  FigPos=figposition([2.5 68.5 70 25]);  AxisProperties=off  XUnits=Hertz  XRange=[-Fs/2...Fs/2]  InheritXIncr=off  XIncr=1e-8  XLabel=Time  YUnits=Magnitude  YLabel=Magnitude, dB  LineProperties=off  LineStyles=--  LineColors=m
      settings: YMin=-80.906815143504  YMax=-25.7732682054945
  Sum : Sum  Inputs=|++  SaturateOnIntegerOverflow=on  InputSameDT=on
  Sum1 : Sum  Inputs=|++  SaturateOnIntegerOverflow=on  InputSameDT=on
  Timing Diagram : dspsnks4/Vector Scope  ScopeProperties=off  Domain=User-defined  HorizSpan=1  DisplayProperties=off  AxisGrid=on  Memory=off  FrameNumber=on  AxisLegend=on  AxisZoom=off  OpenScopeAtSimStart=on  OpenScopeImmediately=off  FigPos=figposition([2.5 37.5 70 25]);  AxisProperties=off  XUnits=Hertz  XRange=[0...Fs/2]  InheritXIncr=off  XIncr=125*1e-8  XLabel=Time (s)  YUnits=dB  YLabel=Amplitude  LineProperties=off  LineStyles=-|-  LineColors=[0 0 1]|[1 0 0]
      settings: YMin=-0.525  YMax=1.05
  Transpose1 : dspmtrx3/Transpose  Hermitian=off  overflowFlag=on
  Transpose2 : dspmtrx3/Transpose  Hermitian=off  overflowFlag=on
  dB Conversion1 : dspmathops/dB Conversion  dBtype=dB  intype=Power  R=1  fuzz=on
  enable : dspsrcs4/Signal From Workspace  X=[1 0 0 0 0 0]  Ts=625e-6  nsamps=1  OutputAfterFinalValue=Cyclic repetition
  wires:
  DSP Constant/1 -> Sum1/2
  Sum1/1 -> Downsample1/1
  Marker/1(Tx) -> Sum1/1
  Buffer1/1 -> Sum/1
  Constant2/1 -> Sum/2
  Matrix Concatenation/1 -> Multiport Selector/1
  Relational Operator1/1 -> Matrix Concatenation/1
  Sum/1 -> Matrix Concatenation/2
  Downsample1/1 -> Buffer1/1
  Multiport Selector/3 -> Matrix Concatenation1/3  "Slots"
  enable/1 -> Marker/Enable
  Multiport Selector/2 -> Matrix Concatenation1/2  "802.11b Tx"
  Multiport Selector/1 -> Matrix Concatenation1/1  "Bluetooth Tx"
  Matrix Concatenation2/1 -> Downsample/1
  In1/1 -> Matrix Concatenation2/1
  In2/1 -> Matrix Concatenation2/2
  Buffer/1 -> Relational Operator1/1
  Constant1/1 -> Relational Operator1/2
  Transpose2/1 -> dB Conversion1/1
  Transpose1/1 -> Mean/1
  Mean/1 -> Transpose2/1
  Reshape/1 -> Short-Time FFT1/1
  In3/1 -> Reshape/1
  Matrix Concatenation1/1 -> Timing Diagram/1
  Short-Time FFT1/1 -> Transpose1/1
  dB Conversion1/1 -> Spectrum Plot/1  "ISM Band Spectrum"
  Downsample/1 -> Abs/1
  Abs/1 -> Buffer/1

== system bluetooth_voice/Slave Receiver/CVSD Decode ==
  In1 : Inport  LatchInput=off
  Enable : EnablePort
  Delay : dspsigops/Delay  dly_unit=Samples  delay=1  ic_detail=on  dif_ic_for_ch=off  dif_ic_for_dly=off  ic=10  reset_popup=None
  Digital Filter Design : dsparch4/Digital Filter Design
  Gain1 : Gain  Gain=1/32768  SaturateOnIntegerOverflow=on
  Unipolar to Bipolar Converter : commutil2/Unipolar to Bipolar Converter  M=2  polarity=Negative
  Update accum : Subsystem  PropExecContextAcrossSSBoundary=on
  Update runner : Subsystem  PropExecContextAcrossSSBoundary=on
  Update stepsize : Subsystem  PropExecContextAcrossSSBoundary=on
  accum : dspsigops/Delay  dly_unit=Samples  delay=1  ic_detail=on  dif_ic_for_ch=off  dif_ic_for_dly=off  ic=0  reset_popup=None
  stepsize : dspsigops/Delay  dly_unit=Samples  delay=1  ic_detail=on  dif_ic_for_ch=off  dif_ic_for_dly=off  ic=min_step  reset_popup=None
  Out2 : Outport
  wires:
  In1/1 -> Unipolar to Bipolar Converter/1  "u"
  accum/1 -> Update accum/3(accum(n))  "accum(n)"
  Delay/1 -> Update runner/2(runner(n))  "runner(n)"
  Update runner/1(runner(n+1)) -> Update stepsize/1(runner(n+1)), Delay/1  "runner(n+1)"
  stepsize/1 -> Update stepsize/2(stepsize(n))  "stepsize(n)"
  Update stepsize/1(stepsize(n+1)) -> Update accum/1(stepsize(n+1)), stepsize/1  "stepsize(n+1)"
  Update accum/1(accum(n+1)) -> Gain1/1, accum/1  "accum(n+1)"
  Unipolar to Bipolar Converter/1 -> Update accum/2(u), Update runner/1(u)  "u"
  Digital Filter Design/1 -> Out2/1
  Gain1/1 -> Digital Filter Design/1

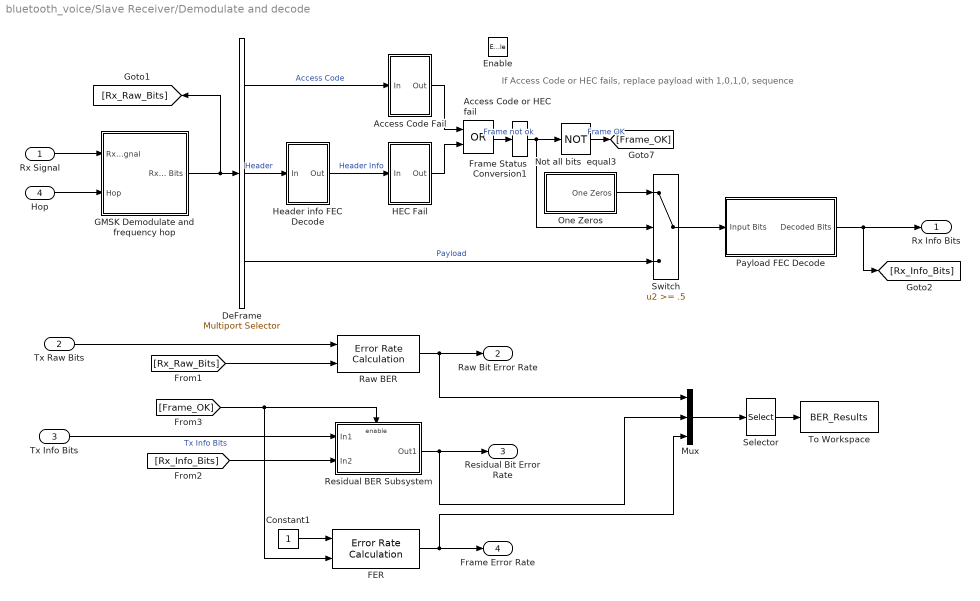
== system bluetooth_voice/Slave Receiver/Demodulate and decode ==
  note: If Access Code or HEC fails,
      | replace payload with 1,0,1,0, sequence
  Rx Signal : Inport  LatchInput=off
  Tx Raw Bits : Inport  Port=2  LatchInput=off
  Tx Info Bits : Inport  Port=3  LatchInput=off
  Hop : Inport  Port=4  SampleTime=Slot_Ts  LatchInput=off
  Enable : EnablePort
  Access Code Fail : Subsystem  PropExecContextAcrossSSBoundary=on
  Access Code or HEC fail : Logic  Operator=OR
  Constant1 : Constant
  DeFrame : dspindex/Multiport Selector  rowsOrCols=Rows  idxCellArray="{  1:72, 73:126,127:366}"  idxErrMode=Clip Index
  FER : commsink2/Error Rate Calculation  N=0  st_delay=0  cp_mode=Entire frame  subframe=[]  PMode=Port  WsName=ErrorVec  RsMode2=off  stop=on  numErr=100  maxBits=1e6
  Frame Status Conversion1 : dspsigattribs/Frame Status Conversion  growRefPort=off  outframe=Sample-based
  GMSK Demodulate and frequency hop : Subsystem  PropExecContextAcrossSSBoundary=on
  HEC Fail : Subsystem  PropExecContextAcrossSSBoundary=on
  Header info FEC Decode : Subsystem  PropExecContextAcrossSSBoundary=on
  Mux : Mux  Inputs=3
  Not all bits  equal3 : Logic  Operator=NOT  Inputs=1
  One Zeros : Subsystem  PropExecContextAcrossSSBoundary=on
  Payload FEC Decode : Subsystem  PropExecContextAcrossSSBoundary=on
  Raw BER : commsink2/Error Rate Calculation  N=0  st_delay=0  cp_mode=Entire frame  subframe=[]  PMode=Port  WsName=ErrorVec  RsMode2=off  stop=off  numErr=100  maxBits=1e6
  Residual BER Subsystem : Subsystem  TreatAsAtomicUnit=on  PropExecContextAcrossSSBoundary=on
  Selector : Selector  Elements=[1 4 7]  InputPortWidth=9
  Switch : Switch  Threshold=.5  InputSameDT=on
  To Workspace : ToWorkspace  VariableName=BER_Results  SampleTime=-1  SaveFormat=Array
      settings: MaxDataPoints=1
  Rx Info Bits : Outport  InitialOutput=0
  Raw Bit Error Rate : Outport  Port=2  InitialOutput=0
  Residual Bit Error Rate : Outport  Port=3  InitialOutput=0
  Frame Error Rate : Outport  Port=4  InitialOutput=0
  wires:
  Hop/1 -> GMSK Demodulate and frequency hop/2(Hop)
  Rx Signal/1 -> GMSK Demodulate and frequency hop/1(Rx Signal)
  Switch/1 -> Payload FEC Decode/1(Input Bits)
  Not all bits  equal3/1 -> [Frame_OK]  "Frame OK"
  Frame Status Conversion1/1 -> Not all bits  equal3/1, Switch/2
  HEC Fail/1(Out) -> Access Code or HEC fail/2
  Header info FEC Decode/1(Out) -> HEC Fail/1(In)  "Header Info"
  Access Code Fail/1(Out) -> Access Code or HEC fail/1
  Access Code or HEC fail/1 -> Frame Status Conversion1/1  "Frame not ok"
  DeFrame/2 -> Header info FEC Decode/1(In)  "Header"
  One Zeros/1(One Zeros) -> Switch/1
  DeFrame/1 -> Access Code Fail/1(In)  "Access Code"
  DeFrame/3 -> Switch/3  "Payload"
  Tx Info Bits/1 -> Residual BER Subsystem/1(In1)  "Tx Info Bits"
  [Rx_Info_Bits] -> Residual BER Subsystem/2(In2)
  Constant1/1 -> FER/1
  Selector/1 -> To Workspace/1
  Mux/1 -> Selector/1
  Raw BER/1 -> Mux/1, Raw Bit Error Rate/1
  Tx Raw Bits/1 -> Raw BER/1
  FER/1 -> Mux/3, Frame Error Rate/1
  [Frame_OK] -> FER/2, Residual BER Subsystem/Enable
  Residual BER Subsystem/1(Out1) -> Mux/2, Residual Bit Error Rate/1
  Payload FEC Decode/1(Decoded Bits) -> [Rx_Info_Bits], Rx Info Bits/1
  [Rx_Raw_Bits] -> Raw BER/2
  GMSK Demodulate and frequency hop/1(Rx Raw Bits) -> DeFrame/1, [Rx_Raw_Bits]

== system bluetooth_voice/AWGN/Subsystem/Add noise ==
  In1 : Inport  LatchInput=off
  Action Port : ActionPort  ActionType=else
  AWGN Channel1 : commchan2/AWGN Channel  seed=seed  noiseMode="Signal to noise ratio  (Es/No)"  EbNodB=10  EsNodB=EsNo  SNRdB=10  bitsPerSym=1  Ps=Power  Tsym=Symbol_Period  variance=1
  Out1 : Outport
  wires:
  In1/1 -> AWGN Channel1/1
  AWGN Channel1/1 -> Out1/1

== system bluetooth_voice/AWGN/Subsystem/Pass Through ==
  In1 : Inport  LatchInput=off
  Action Port : ActionPort  ActionType=then
  Out1 : Outport
  wires:
  In1/1 -> Out1/1

== system bluetooth_voice/Master Transmitter/CVSD Encode/Set any 0's to 1's ==
  In1 : Inport  LatchInput=off
  If : If  IfExpression=u1 ==0
  Merge : Merge
  Pass through : Subsystem  TreatAsAtomicUnit=on  PropExecContextAcrossSSBoundary=on
  Set to 1 : Subsystem  TreatAsAtomicUnit=on  PropExecContextAcrossSSBoundary=on
  Out1 : Outport
  wires:
  If/1 -> Set to 1/Action
  In1/1 -> Pass through/1(In1), If/1
  If/2 -> Pass through/Action
  Set to 1/1(1) -> Merge/1
  Pass through/1(Out1=In1) -> Merge/2
  Merge/1 -> Out1/1  "y"

== system bluetooth_voice/Master Transmitter/CVSD Encode/Update accum ==
  stepsize(n+1) : Inport  LatchInput=off
  y : Inport  Port=2  LatchInput=off
  accum(n) : Inport  Port=3  LatchInput=off
  Gain : Gain  Gain=accum_decay  SaturateOnIntegerOverflow=on
  Product : Product  SaturateOnIntegerOverflow=on  InputSameDT=on
  Saturation : Saturate  UpperLimit=pos_accum_max  LowerLimit=neg_accum_max
  Sum1 : Sum  Inputs=|++  SaturateOnIntegerOverflow=on  InputSameDT=on
  accum(n+1) : Outport
  wires:
  Gain/1 -> Saturation/1
  Product/1 -> Sum1/1  "y*stepsize"
  Sum1/1 -> Gain/1
  stepsize(n+1)/1 -> Product/1
  y/1 -> Product/2
  accum(n)/1 -> Sum1/2
  Saturation/1 -> accum(n+1)/1

== system bluetooth_voice/Master Transmitter/CVSD Encode/Update runner ==
  y : Inport  LatchInput=off
  runner(n) : Inport  Port=2  LatchInput=off
  Bitwise Logical Operator : simulink/Logic and Bit Operations/Bitwise Operator  logicop=AND  UseBitMask=on  BitMask=15  BitMaskRealWorld=Stored Integer
  Data Type Conversion : DataTypeConversion  OutDataTypeMode=uint16  SaturateOnIntegerOverflow=on  RndMeth=Zero
  Data Type Conversion1 : DataTypeConversion  OutDataTypeMode=double  SaturateOnIntegerOverflow=on  RndMeth=Zero
  Fcn : Fcn  Expr=u==1
  Gain : Gain  Gain=2  SaturateOnIntegerOverflow=on
  Sum1 : Sum  Inputs=|++  SaturateOnIntegerOverflow=on  InputSameDT=on
  runner(n+1) : Outport
  wires:
  Gain/1 -> Sum1/2  "2*runner"
  Fcn/1 -> Sum1/1  "y==1"
  Sum1/1 -> Data Type Conversion/1
  Data Type Conversion/1 -> Bitwise Logical Operator/1
  y/1 -> Fcn/1
  Bitwise Logical Operator/1 -> Data Type Conversion1/1
  runner(n)/1 -> Gain/1
  Data Type Conversion1/1 -> runner(n+1)/1

== system bluetooth_voice/Master Transmitter/CVSD Encode/Update stepsize ==
  runner(n+1) : Inport  LatchInput=off
  stepsize(n) : Inport  Port=2  LatchInput=off
  If : If  IfExpression=(u1 == 0) | (u1== 15)
  Merge1 : Merge
  Update : Subsystem  TreatAsAtomicUnit=on  PropExecContextAcrossSSBoundary=on
  Update1 : Subsystem  TreatAsAtomicUnit=on  PropExecContextAcrossSSBoundary=on
  stepsize(n+1) : Outport
  wires:
  If/2 -> Update1/Action
  If/1 -> Update/Action  "(runner == 0) | (runner == 15)"
  Update/1(stepsize(n+1)) -> Merge1/1
  stepsize(n)/1 -> Update1/1(stepsize), Update/1(stepsize)
  Update1/1(stepsize(n+1)) -> Merge1/2
  runner(n+1)/1 -> If/1
  Merge1/1 -> stepsize(n+1)/1

== system bluetooth_voice/Master Transmitter/Encode and modulate/GFSK Modulate and frequency hop ==
  Tx Raw Bits : Inport  LatchInput=off
  Hop : Inport  Port=2  LatchInput=off
  Frame Status Conversion : dspsigattribs/Frame Status Conversion  growRefPort=off  outframe=Frame-based
  Free Space Path Loss : commrflib2/Free Space Path Loss  mode=Decibels  dB=30  d=0.100  fc=1920
  GFSK Modulation : commdigbbndcpm2/CPM Modulator Baseband  Mnum=2  inputType=Bit  mappingType=Binary  modIdx=0.32  pulseShape=Gaussian  BT=0.5  mainLobePulseLength=1  rollOff=0.2  pulseLength=1  preHistory=1  phaseOffset=0  samplesPerSymbol=100
  "Generate 79 possible carriers -39MHz to 39MHz " : commdigbbndfm2/M-FSK Modulator Baseband  M=79  InType=Integer  Enc=Binary  freqSep=1e6  phaseType=Continuous  numSamp=6.25e4
  Mask to turn off transmitter after data finished : Gain  Gain=[ones(36600,1);zeros(62500-36600,1)]  SaturateOnIntegerOverflow=on
  Product3 : Product  SaturateOnIntegerOverflow=on  InputSameDT=on
  Zero Pad to fill slot : dspsigops/Zero Pad  padSigAt=End  zpadAlong=Columns  padNumOutRowsSpecMethod=User-specified  numOutRows=625  padNumOutColsSpecMethod=User-specified  numOutCols=1  trunc_flag=None
  Tx SIgnal : Outport
  wires:
  Product3/1 -> Mask to turn off transmitter after data finished/1
  Mask to turn off transmitter after data finished/1 -> Free Space Path Loss/1
  Zero Pad to fill slot/1 -> GFSK Modulation/1
  Frame Status Conversion/1 -> "Generate 79 possible carriers -39MHz to 39MHz "/1
  "Generate 79 possible carriers -39MHz to 39MHz "/1 -> Product3/2
  GFSK Modulation/1 -> Product3/1
  Tx Raw Bits/1 -> Zero Pad to fill slot/1
  Free Space Path Loss/1 -> Tx SIgnal/1
  Hop/1 -> Frame Status Conversion/1

== system bluetooth_voice/Master Transmitter/Encode and modulate/Header Info ==
  Header3 : dspsrcs4/DSP Constant  Value=Slave_Address  SampleMode=Discrete  discreteOutput=Frame-based  continuousOutput=Sample-based  sampTime=Slot_Ts  framePeriod=Slot_Ts  dataType=Inherit from 'Constant value'  isSigned=on  wordLen=16  udDataType=sfix(16)  fracBitsMode=Best precision  numFracBits=15  InterpretAs1D=off  Ts=Slot_Ts  FramebasedOutput=on
  Header4 : dspsrcs4/DSP Constant  Value=Packet_Type  SampleMode=Discrete  discreteOutput=Frame-based  continuousOutput=Sample-based  sampTime=Slot_Ts  framePeriod=Slot_Ts  dataType=Inherit from 'Constant value'  isSigned=on  wordLen=16  udDataType=sfix(16)  fracBitsMode=Best precision  numFracBits=15  InterpretAs1D=off  Ts=Slot_Ts  FramebasedOutput=on
  Header5 : dspsrcs4/DSP Constant  Value=Flow_Control  SampleMode=Discrete  discreteOutput=Frame-based  continuousOutput=Sample-based  sampTime=Slot_Ts  framePeriod=Slot_Ts  dataType=Inherit from 'Constant value'  isSigned=on  wordLen=16  udDataType=sfix(16)  fracBitsMode=Best precision  numFracBits=15  InterpretAs1D=off  Ts=Slot_Ts  FramebasedOutput=on
  Header6 : dspsrcs4/DSP Constant  Value=ARQ  SampleMode=Discrete  discreteOutput=Frame-based  continuousOutput=Sample-based  sampTime=Slot_Ts  framePeriod=Slot_Ts  dataType=Inherit from 'Constant value'  isSigned=on  wordLen=16  udDataType=sfix(16)  fracBitsMode=Best precision  numFracBits=15  InterpretAs1D=off  Ts=Slot_Ts  FramebasedOutput=on
  Header7 : dspsrcs4/DSP Constant  Value=Sequence  SampleMode=Discrete  discreteOutput=Frame-based  continuousOutput=Sample-based  sampTime=Slot_Ts  framePeriod=Slot_Ts  dataType=Inherit from 'Constant value'  isSigned=on  wordLen=16  udDataType=sfix(16)  fracBitsMode=Best precision  numFracBits=15  InterpretAs1D=off  Ts=Slot_Ts  FramebasedOutput=on
  Matrix Concatenation1 : simulink/Math Operations/Matrix Concatenation  numInports=5  catMethod=Vertical
  Out : Outport
  wires:
  Header3/1 -> Matrix Concatenation1/1  "Slave address"
  Header4/1 -> Matrix Concatenation1/2  "Packet type"
  Header5/1 -> Matrix Concatenation1/3  "Flow control"
  Header6/1 -> Matrix Concatenation1/4  "ARQ"
  Header7/1 -> Matrix Concatenation1/5  "Sequence"
  Matrix Concatenation1/1 -> Out/1  "Header Info"

== system bluetooth_voice/Master Transmitter/Payload FEC Encode/FEC HV1 ==
  In : Inport  LatchInput=off
  Enable : EnablePort
  Buffer : dspbuff3/Buffer  N=80  V=0  ic=0
  FEC : dspsigops/Repeat  N=3  ic=0  mode=Maintain input frame rate
  Sample Tx_Ts1 : ZeroOrderHold  SampleTime=Slot_Ts
  Sample Tx_Ts2 : ZeroOrderHold  SampleTime=Slot_Ts
  Zero Pad : dspsigops/Zero Pad  padSigAt=End  zpadAlong=Columns  padNumOutRowsSpecMethod=User-specified  numOutRows=240  padNumOutColsSpecMethod=User-specified  numOutCols=1  trunc_flag=None
  FEC'd : Outport
  Bits : Outport  Port=2
  wires:
  In/1 -> Buffer/1
  FEC/1 -> Sample Tx_Ts1/1
  Sample Tx_Ts1/1 -> FEC'd/1
  Zero Pad/1 -> Sample Tx_Ts2/1
  Sample Tx_Ts2/1 -> Bits/1
  Buffer/1 -> FEC/1, Zero Pad/1
